simulink model "Modelo_irradiancia_parcial"  (R2021a)
settings: Solver=VariableStepAuto  StartTime=0.0  StopTime=50  FixedStep=Ts_Power  MaxStep=1e-6  RelTol=1e-4
StopFcn:
  | VI_generator()
values from neighbouring files (symbols this model uses):
  Ir = Irmin+(Irmax-Irmin).*rand(nmodulos,1)    [Data_generation.m]
  T = Ta+G*((Tonc-20)/800)    [Data_generation.m]
undefined symbols (not defined in the file or in its folder): Ts_Power
libraries: spsPVArrayLib x10, spsDiodeLib x5, spsCurrentMeasurementLib x1, spsControlledVoltageSourceLib x1, simulink x1, spsVoltageMeasurementLib x1, spspowerguiLib x1
settings Model: Creator=MathWorks  LastModifiedBy=Guillermo
settings SolverCC: AlgebraicLoopSolver=LineSearch
settings DataIOCC: LimitDataPoints=on  SaveFormat=Array  SignalLoggingSaveFormat=ModelDataLogs  ReturnWorkspaceOutputs=off
settings OptimizationCC: ExpressionDepthLimit=2147483647  LifeSpan=inf
settings DebuggingCC: UnderspecifiedInitializationDetection=Classic  MergeDetectMultiDrivingBlocksExec=none  SolverPrmCheckMsg=warning  FcnCallInpInsideContextMsg=warning  AllowSymbolicDim=off  StateNameClashWarn=warning  SFUnexpectedBacktrackingDiag=warning  SFNoUnconditionalDefaultTransitionDiag=warning  SFExecutionAtInitializationDiag=none  SFMachineParentedDataDiag=warning  ArithmeticOperatorsInVariantConditions=warning
settings HardwareCC: ProdBitPerPointer=32  ProdBitPerSizeT=32  ProdBitPerPtrDiffT=32  ProdLargestAtomicFloat=None  ProdIntDivRoundTo=Undefined  ProdEndianess=Unspecified  ProdWordSize=32  ProdHWDeviceType=32-bit Generic
settings ModelReferenceCC: PropagateSignalLabelsOutOfModel=off
settings SFSimCC: SimUseLocalCustomCode=off  CustomCodeUndefinedFunction=UseInterfaceOnly
settings RTWCC: RTWUseLocalCustomCode=off
settings CodeAppCC: StateflowObjectComments=on
settings GRTTargetCC: TargetLangStandard=C89/C90 (ANSI)  CombineOutputUpdateFcns=off  GRTInterface=on
settings ConfigComp: CovMetricSettings=dw  CovSaveCumulativeToWorkspaceVar=on  CovSaveSingleToWorkspaceVar=on  CovExternalEMLEnable=off  CovSFcnEnable=off
settings SimscapeCC: SimscapeNormalizeSystem=off

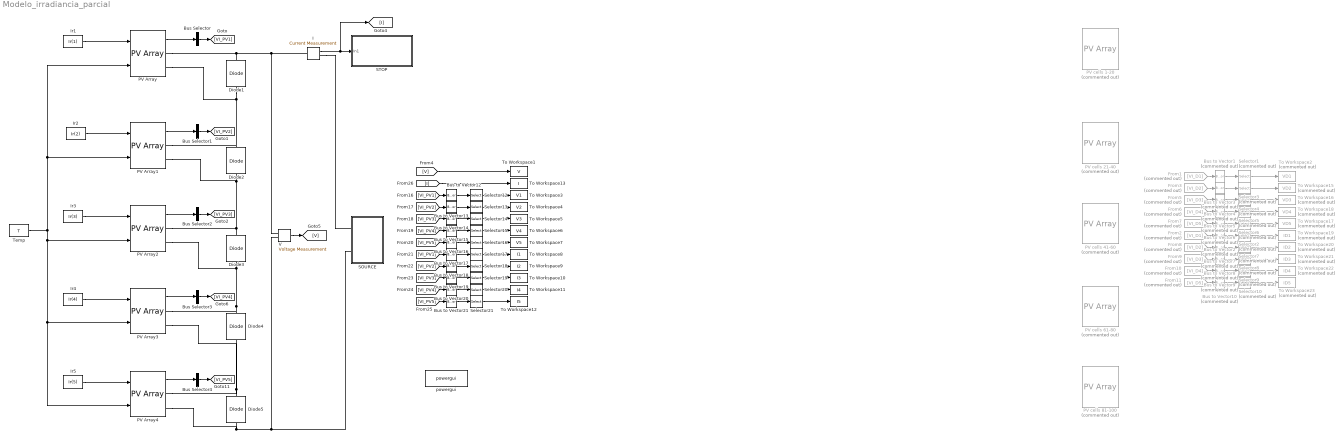
== system Modelo_irradiancia_parcial ==
  Bus Selector{,1..4} (5 alike) : BusSelector  OutputSignals=V_PV,I_PV  OutputAsBus=on
  Bus to Vector{1..10} (10 alike) : BusToVector  Commented=on
  Bus to Vector{12..21} (10 alike) : BusToVector
  Diode{1..5} (5 alike) : spsDiodeLib/Diode  Ron=0.001  Lon=0  Vf=0.7  IC=0  UseSnubber=off  Rs=1e5*inf  Cs=inf  Measurements=off
  From1 : From  Commented=on  GotoTag=VI_D1
  From10 : From  Commented=on  GotoTag=VI_D4
  From11 : From  Commented=on  GotoTag=VI_D5
  From2 : From  Commented=on  GotoTag=VI_D1
  From3 : From  Commented=on  GotoTag=VI_D2
  From5 : From  Commented=on  GotoTag=VI_D3
  From6 : From  Commented=on  GotoTag=VI_D4
  From7 : From  Commented=on  GotoTag=VI_D5
  From8 : From  Commented=on  GotoTag=VI_D2
  From9 : From  Commented=on  GotoTag=VI_D3
  I : spsCurrentMeasurementLib/Current Measurement  PhasorSimulation=off  OutputType=Complex  PSBequivalent=0
  Ir1 : Constant  Value=Ir(1)
  Ir2 : Constant  Value=Ir(2)
  Ir3 : Constant  Value=Ir(3)
  Ir4 : Constant  Value=Ir(4)
  Ir5 : Constant  Value=Ir(5)
  PV Array{,1..4} (5 alike) : spsPVArrayLib/PV Array  Npar=1  Nser=1  PlotType=array @ 25 deg.C & specified irradiances  S_vec="[ 1000  500  100 ]"  Temp_C_vec="[ 45 25  ]"  ModuleName=SunPower SPR-305E-WHT-D  PlotWhenSelected=off  Pm=305.226  Ncell=96  Voc=64.2  Isc=5.96  Vm=54.7  Im=5.58  beta_Voc_pc=-0.2727  alpha_Isc_pc=0.061745  beta_Voc=-0.17507  alpha_Isc=0.00368  IL=5.9657  I0=6.3076e-12  nI=0.94489  Rsh=393.2054  Rs=0.37428  RobustModel=off  RobustCellTemperature=313.3991  BAL=on  Tc=1e-4  Tfilter=5e-5
  PV cells 1-20 : spsPVArrayLib/PV Array  Commented=on  Npar=2  Nser=10  PlotType=array @ 25 deg.C & specified irradiances  S_vec="[ 1000  500  100 ]"  Temp_C_vec="[ 45 25  ]"  ModuleName=User-defined  PlotWhenSelected=off  Pm=5.4719  Ncell=1  Voc=0.682  Isc=9.864  Vm=0.581  Im=9.418  beta_Voc_pc=-0.28  alpha_Isc_pc=0.04  beta_Voc=-0.0019096  alpha_Isc=0.0039456  IL=9.8771  I0=1.4094e-11  nI=0.97343  Rsh=11.5037  Rs=0.0023503  RobustModel=off  RobustCellTemperature=25  BAL=on  Tc=1e-5  Tfilter=5e-5
  PV cells 21-40 : spsPVArrayLib/PV Array  Commented=on  Npar=2  Nser=10  PlotType=array @ 25 deg.C & specified irradiances  S_vec="[ 1000  500  100 ]"  Temp_C_vec="[ 45 25  ]"  ModuleName=User-defined  PlotWhenSelected=off  Pm=5.4719  Ncell=1  Voc=0.682  Isc=9.864  Vm=0.581  Im=9.418  beta_Voc_pc=-0.28  alpha_Isc_pc=0.04  beta_Voc=-0.0019096  alpha_Isc=0.0039456  IL=9.8771  I0=1.4094e-11  nI=0.97343  Rsh=11.5037  Rs=0.0023503  RobustModel=off  RobustCellTemperature=25  BAL=on  Tc=1e-5  Tfilter=5e-5
  PV cells 41-60 : spsPVArrayLib/PV Array  Commented=on  Npar=2  Nser=10  PlotType=array @ 25 deg.C & specified irradiances  S_vec="[ 1000  500  100 ]"  Temp_C_vec="[ 45 25  ]"  ModuleName=User-defined  PlotWhenSelected=off  Pm=5.4719  Ncell=1  Voc=0.682  Isc=9.864  Vm=0.581  Im=9.418  beta_Voc_pc=-0.28  alpha_Isc_pc=0.04  beta_Voc=-0.0019096  alpha_Isc=0.0039456  IL=9.8771  I0=1.4094e-11  nI=0.97343  Rsh=11.5037  Rs=0.0023503  RobustModel=off  RobustCellTemperature=25  BAL=on  Tc=1e-5  Tfilter=5e-5
  PV cells 61-80 : spsPVArrayLib/PV Array  Commented=on  Npar=2  Nser=10  PlotType=array @ 25 deg.C & specified irradiances  S_vec="[ 1000  500  100 ]"  Temp_C_vec="[ 45 25  ]"  ModuleName=User-defined  PlotWhenSelected=off  Pm=5.4719  Ncell=1  Voc=0.682  Isc=9.864  Vm=0.581  Im=9.418  beta_Voc_pc=-0.28  alpha_Isc_pc=0.04  beta_Voc=-0.0019096  alpha_Isc=0.0039456  IL=9.8771  I0=1.4094e-11  nI=0.97343  Rsh=11.5037  Rs=0.0023503  RobustModel=off  RobustCellTemperature=25  BAL=on  Tc=1e-5  Tfilter=5e-5
  PV cells 81-100 : spsPVArrayLib/PV Array  Commented=on  Npar=2  Nser=10  PlotType=array @ 25 deg.C & specified irradiances  S_vec="[ 1000  500  100 ]"  Temp_C_vec="[ 45 25  ]"  ModuleName=User-defined  PlotWhenSelected=off  Pm=5.4719  Ncell=1  Voc=0.682  Isc=9.864  Vm=0.581  Im=9.418  beta_Voc_pc=-0.28  alpha_Isc_pc=0.04  beta_Voc=-0.0019096  alpha_Isc=0.0039456  IL=9.8771  I0=1.4094e-11  nI=0.97343  Rsh=11.5037  Rs=0.0023503  RobustModel=off  RobustCellTemperature=25  BAL=on  Tc=1e-5  Tfilter=5e-5
  SOURCE : Subsystem
  STOP : Subsystem
  Selector{1,3..6} (5 alike) : Selector  Commented=on  InputPortWidth=2  IndexOptions=Index vector (dialog)  Indices=[1]  OutputSizes=1
  Selector{2,7..10} (5 alike) : Selector  Commented=on  InputPortWidth=2  IndexOptions=Index vector (dialog)  Indices=2  OutputSizes=1
  Selector{12..16} (5 alike) : Selector  InputPortWidth=2  IndexOptions=Index vector (dialog)  Indices=[1]  OutputSizes=1
  Selector{17..21} (5 alike) : Selector  InputPortWidth=2  IndexOptions=Index vector (dialog)  Indices=2  OutputSizes=1
  Temp : Constant  Value=T
  To Workspace1 : ToWorkspace  VariableName=V  SampleTime=1e-3
  To Workspace10 : ToWorkspace  VariableName=I3  SampleTime=1e-3
  To Workspace11 : ToWorkspace  VariableName=I4  SampleTime=1e-3
  To Workspace12 : ToWorkspace  VariableName=I5  SampleTime=1e-3
  To Workspace13 : ToWorkspace  VariableName=I  SampleTime=1e-3
  To Workspace15 : ToWorkspace  Commented=on  VariableName=VD2  SampleTime=1e-3
  To Workspace16 : ToWorkspace  Commented=on  VariableName=VD3  SampleTime=1e-3
  To Workspace17 : ToWorkspace  Commented=on  VariableName=VD5  SampleTime=1e-3
  To Workspace18 : ToWorkspace  Commented=on  VariableName=VD4  SampleTime=1e-3
  To Workspace19 : ToWorkspace  Commented=on  VariableName=ID1  SampleTime=1e-3
  To Workspace2 : ToWorkspace  Commented=on  VariableName=VD1  SampleTime=1e-3
  To Workspace20 : ToWorkspace  Commented=on  VariableName=ID2  SampleTime=1e-3
  To Workspace21 : ToWorkspace  Commented=on  VariableName=ID3  SampleTime=1e-3
  To Workspace22 : ToWorkspace  Commented=on  VariableName=ID4  SampleTime=1e-3
  To Workspace23 : ToWorkspace  Commented=on  VariableName=ID5  SampleTime=1e-3
  To Workspace3 : ToWorkspace  VariableName=V1  SampleTime=1e-3
  To Workspace4 : ToWorkspace  VariableName=V2  SampleTime=1e-3
  To Workspace5 : ToWorkspace  VariableName=V3  SampleTime=1e-3
  To Workspace6 : ToWorkspace  VariableName=V4  SampleTime=1e-3
  To Workspace7 : ToWorkspace  VariableName=V5  SampleTime=1e-3
  To Workspace8 : ToWorkspace  VariableName=I1  SampleTime=1e-3
  To Workspace9 : ToWorkspace  VariableName=I2  SampleTime=1e-3
  V : spsVoltageMeasurementLib/Voltage Measurement  PhasorSimulation=off  OutputType=Complex  PSBequivalent=0
  powergui : spspowerguiLib/powergui  Priority=1  SimulationMode=Continuous  SampleTime=Ts_Power*0 + 20e-6  frequency=60  Iterations=50  frequencyindice=0  Pbase=100e6  ErrMax=1e-4  UnitsV=kV  UnitsW=MW  buscounter=0  FunctionMessages=off  echomessages=off  EnableUseOfTLC=off  CurrentSourceSwitches=on  DisableSnubberDevices=on  DisableRonSwitches=off  DisableVfSwitches=off  DisplayEquations=off  AutomaticDiscreteSolvers=off  SolverType=Tustin/Backward Euler (TBE)  Interpol=off  ExternalGateDelay=off  methode=off  Ts=0  x0status=blocks  SPID=off  SwTol=0  HookPort=off  NonlinearTolerance=1e-4  nMaxIteration=100  ContinueOnMaxIteration=off  RestoreLinks=warning  ResistiveCurrentMeasurement=off  Frange=[0:2:500]  Ylog=off  Xlog=on  ShowGrid=off  save=off  variable=ZData  structure=0  ZoomFFT=on  StartTime=0.0  cycles=1  DisplayStyle=1  fundamental=60  FreqAxis=off  MaxFrequency=1000  frequencyindicesteady=1  RmsSteady=1  display=off
  wires:
  V/1 -> [V]
  PV Array/1 -> Bus Selector/1
  Bus Selector/1 -> [VI_PV1]
  Bus Selector1/1 -> [VI_PV2]
  PV Array1/1 -> Bus Selector1/1
  Bus Selector2/1 -> [VI_PV3]
  PV Array2/1 -> Bus Selector2/1
  Ir3/1 -> PV Array2/1
  Ir2/1 -> PV Array1/1
  Ir1/1 -> PV Array/1
  Ir4/1 -> PV Array3/1
  PV Array3/1 -> Bus Selector3/1
  Bus Selector3/1 -> [VI_PV4]
  Ir5/1 -> PV Array4/1
  PV Array4/1 -> Bus Selector4/1
  Bus Selector4/1 -> [VI_PV5]
  Temp/1 -> PV Array1/2, PV Array/2, PV Array2/2, PV Array4/2, PV Array3/2
  Bus to Vector14/1 -> Selector14/1
  [VI_PV1] -> Bus to Vector12/1
  Bus to Vector13/1 -> Selector13/1
  [VI_PV2] -> Bus to Vector13/1
  [VI_PV3] -> Bus to Vector14/1
  Bus to Vector12/1 -> Selector12/1
  [VI_PV4] -> Bus to Vector15/1
  Bus to Vector16/1 -> Selector16/1
  [VI_PV5] -> Bus to Vector16/1
  Bus to Vector15/1 -> Selector15/1
  Selector12/1 -> To Workspace3/1
  Selector16/1 -> To Workspace7/1
  Selector15/1 -> To Workspace6/1
  Selector14/1 -> To Workspace5/1
  Selector13/1 -> To Workspace4/1
  Selector19/1 -> To Workspace10/1
  Selector18/1 -> To Workspace9/1
  Selector21/1 -> To Workspace12/1
  Selector17/1 -> To Workspace8/1
  Bus to Vector17/1 -> Selector17/1
  Bus to Vector18/1 -> Selector18/1
  Bus to Vector20/1 -> Selector20/1
  [VI_PV3] -> Bus to Vector19/1
  [VI_PV1] -> Bus to Vector17/1
  [VI_PV2] -> Bus to Vector18/1
  [VI_PV5] -> Bus to Vector21/1
  [VI_PV4] -> Bus to Vector20/1
  Selector20/1 -> To Workspace11/1
  Bus to Vector21/1 -> Selector21/1
  Bus to Vector19/1 -> Selector19/1
  [I] -> To Workspace13/1
  [V] -> To Workspace1/1
  Bus to Vector1/1 -> Selector1/1
  Selector1/1 -> To Workspace2/1
  From1/1 -> Bus to Vector1/1
  From2/1 -> Bus to Vector2/1
  Bus to Vector2/1 -> Selector2/1
  From3/1 -> Bus to Vector3/1
  Selector3/1 -> To Workspace15/1
  Bus to Vector3/1 -> Selector3/1
  From5/1 -> Bus to Vector4/1
  Selector4/1 -> To Workspace16/1
  Bus to Vector4/1 -> Selector4/1
  From6/1 -> Bus to Vector5/1
  Bus to Vector5/1 -> Selector5/1
  Selector5/1 -> To Workspace18/1
  From7/1 -> Bus to Vector6/1
  Selector6/1 -> To Workspace17/1
  Bus to Vector6/1 -> Selector6/1
  Selector2/1 -> To Workspace19/1
  Bus to Vector7/1 -> Selector7/1
  Selector7/1 -> To Workspace20/1
  From8/1 -> Bus to Vector7/1
  Bus to Vector8/1 -> Selector8/1
  Selector8/1 -> To Workspace21/1
  From9/1 -> Bus to Vector8/1
  Bus to Vector9/1 -> Selector9/1
  Selector9/1 -> To Workspace22/1
  From10/1 -> Bus to Vector9/1
  Bus to Vector10/1 -> Selector10/1
  Selector10/1 -> To Workspace23/1
  From11/1 -> Bus to Vector10/1
  I/1 -> [I], STOP/1(In1)
  connections:
  Diode1/RConn1 -- I/LConn1 -- V/LConn1 -- PV Array/RConn1
  I/RConn1 -- SOURCE/LConn1
  Diode2/LConn1 -- PV Array1/RConn2 -- PV Array2/RConn1 -- Diode3/RConn1
  Diode4/RConn1 -- PV Array3/RConn1 -- PV Array2/RConn2 -- Diode3/LConn1
  PV Array3/RConn2 -- Diode4/LConn1 -- PV Array4/RConn1 -- Diode5/RConn1
  Diode1/LConn1 -- PV Array1/RConn1 -- Diode2/RConn1 -- PV Array/RConn2
  Diode5/LConn1 -- PV Array4/RConn2 -- V/LConn2 -- SOURCE/LConn2

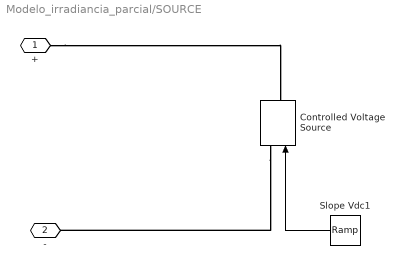
== system Modelo_irradiancia_parcial/SOURCE ==
  Controlled Voltage Source : spsControlledVoltageSourceLib/Controlled Voltage Source  Initialize=on  Source_Type=AC  Amplitude=0  Phase=0  Frequency=0  Measurements=None
  Slope Vdc1 : simulink/Sources/Ramp  slope=2000  start=0  InitialOutput=0
  + : PMIOPort  Side=Left
  - : PMIOPort  Port=2  Side=Left
  wires:
  Slope Vdc1/1 -> Controlled Voltage Source/1
  connections:
  Controlled Voltage Source/LConn1 -- -/RConn1
  +/RConn1 -- Controlled Voltage Source/RConn1

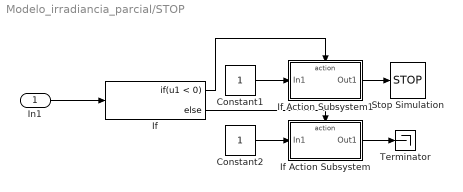
== system Modelo_irradiancia_parcial/STOP ==
  In1 : Inport
  Constant1 : Constant
  Constant2 : Constant
  If : If  IfExpression=u1 < 0
  If Action Subsystem : Subsystem  TreatAsAtomicUnit=on
  If Action Subsystem1 : Subsystem  TreatAsAtomicUnit=on
  Stop Simulation : Stop
  Terminator : Terminator
  wires:
  In1/1 -> If/1
  Constant1/1 -> If Action Subsystem1/1(In1)
  Constant2/1 -> If Action Subsystem/1(In1)
  If Action Subsystem1/1(Out1) -> Stop Simulation/1
  If/1 -> If Action Subsystem1/Action
  If/2 -> If Action Subsystem/Action
  If Action Subsystem/1(Out1) -> Terminator/1

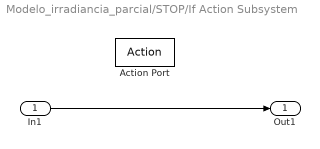
== system Modelo_irradiancia_parcial/STOP/If Action Subsystem ==
  In1 : Inport
  Action Port : ActionPort  ActionPortLabel=else
  Out1 : Outport
  wires:
  In1/1 -> Out1/1

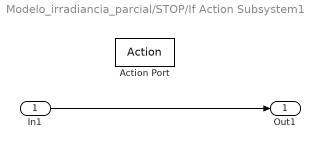
== system Modelo_irradiancia_parcial/STOP/If Action Subsystem1 ==
  In1 : Inport
  Action Port : ActionPort  ActionPortLabel=if(u1 < 0)
  Out1 : Outport
  wires:
  In1/1 -> Out1/1
